simulink model "ModelSquareSubtractive"  (R2018b)
settings: Solver=VariableStepAuto  StartTime=0.0  StopTime=500  MaxStep=0.01  RelTol=1e-4  EnableMultiTasking=on
libraries: fuzblock x1
settings Model: SimulationMode=rapid-accelerator  Creator=DCM  LastModifiedBy=Goncalopinto
settings DataIOCC: LimitDataPoints=on  SaveOutput=off  SaveTime=off
settings OptimizationCC: ExpressionDepthLimit=2147483647  LifeSpan=1
settings DebuggingCC: UnderspecifiedInitializationDetection=Classic  MergeDetectMultiDrivingBlocksExec=none  FcnCallInpInsideContextMsg=warning  AllowSymbolicDim=off  StateNameClashWarn=warning  SFUnexpectedBacktrackingDiag=warning  SFNoUnconditionalDefaultTransitionDiag=warning  SFExecutionAtInitializationDiag=none
settings SFSimCC: SimUseLocalCustomCode=off
settings RTWCC: RTWUseLocalCustomCode=off
settings CodeAppCC: StateflowObjectComments=on
settings GRTTargetCC: TargetLangStandard=C89/C90 (ANSI)  GeneratePreprocessorConditionals=Disable all  CombineOutputUpdateFcns=off  GRTInterface=on

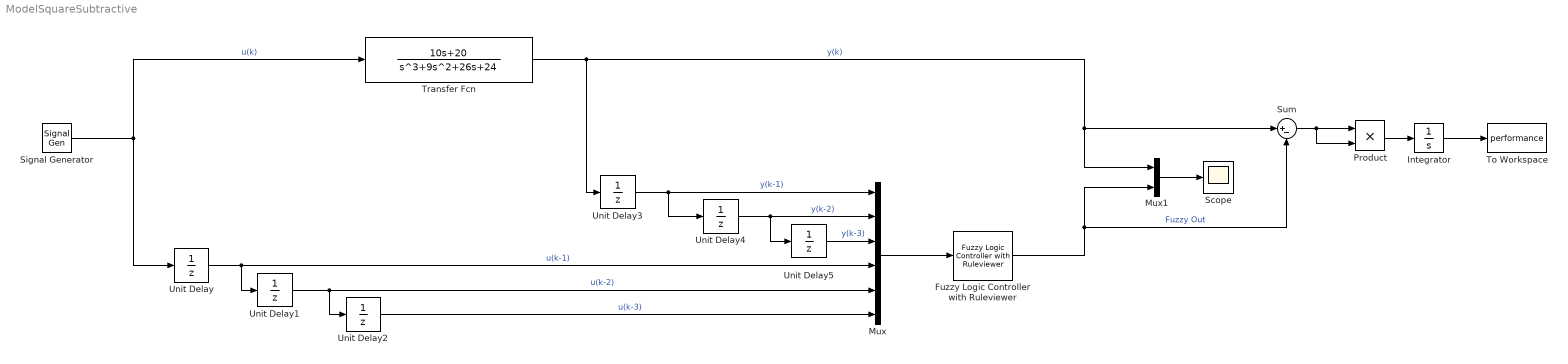
== system ModelSquareSubtractive ==
  Fuzzy Logic Controller with Ruleviewer : fuzblock/Fuzzy Logic  Controller  with Ruleviewer  fismatrix=fis_subtractive  Ts=2
  Integrator : Integrator
  Mux : Mux  Inputs=6
  Mux1 : Mux  Inputs=2
  Product : Product
  Scope : Scope
  Signal Generator : SignalGenerator  WaveForm=square  Frequency=0.1  Units=rad/sec
  Sum : Sum  Inputs=|+-
  To Workspace : ToWorkspace  VariableName=performance  SaveFormat=Structure With Time  SampleTime=-1
  Transfer Fcn : TransferFcn  Numerator=[10 20]  Denominator=[1 9 26 24]
  Unit Delay{,1..5} (6 alike) : UnitDelay  SampleTime=0.0250
  wires:
  Mux1/1 -> Scope/1
  Signal Generator/1 -> Unit Delay/1, Transfer Fcn/1  "u(k)"
  Unit Delay/1 -> Mux/4, Unit Delay1/1  "u(k-1)"
  Unit Delay1/1 -> Mux/5, Unit Delay2/1  "u(k-2)"
  Transfer Fcn/1 -> Unit Delay3/1, Sum/1, Mux1/1  "y(k)"
  Unit Delay3/1 -> Unit Delay4/1, Mux/1  "y(k-1)"
  Unit Delay4/1 -> Mux/2, Unit Delay5/1  "y(k-2)"
  Mux/1 -> Fuzzy Logic Controller with Ruleviewer/1
  Unit Delay2/1 -> Mux/6  "u(k-3)"
  Unit Delay5/1 -> Mux/3  "y(k-3)"
  Fuzzy Logic Controller with Ruleviewer/1 -> Sum/2, Mux1/2  "Fuzzy Out"
  Product/1 -> Integrator/1
  Integrator/1 -> To Workspace/1
  Sum/1 -> Product/2, Product/1
